simulink model "syncbuck_CL"  (Simulink 7.5)
settings: Solver=ode45  StartTime=0.0  StopTime=200e-6  MaxStep=0.1e-6  RelTol=1e-3
libraries: simulink x1
settings Model: Creator=Dragan Maksimovic  LastModifiedBy=Dragan Maksimovic

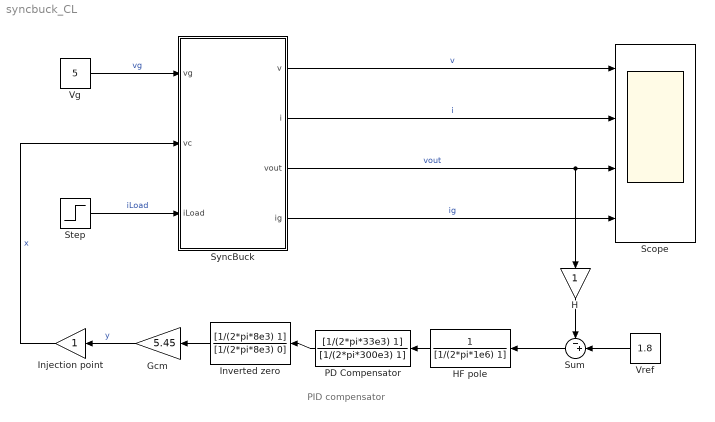
== system syncbuck_CL ==
  note: PID compensator
  " Inverted zero" : TransferFcn  Numerator=[1/(2*pi*8e3) 1]  Denominator=[1/(2*pi*8e3) 0]
  Gcm : Gain  Gain=5.45  ParameterDataType=fixdt(1, 16)  ParameterScaling=2^0  OutDataType=fixdt(1, 16)  OutScaling=2^0
  H : Gain  ParameterDataType=fixdt(1, 16)  ParameterScaling=2^0  OutDataType=fixdt(1, 16)  OutScaling=2^0
  HF pole : TransferFcn  Denominator=[1/(2*pi*1e6) 1]
  Injection point : Gain  ParameterDataType=fixdt(1, 16)  ParameterScaling=2^0  OutDataType=fixdt(1, 16)  OutScaling=2^0
  PD Compensator : TransferFcn  Numerator=[1/(2*pi*33e3) 1]  Denominator=[1/(2*pi*300e3) 1]
  Scope : Scope  NumInputPorts=4
      settings: TimeRange=3.000131492439188e-005  YMin=1.74~-5~1.74~-5  YMax=1.84~10~1.84~10
  Step : Step  Time=120e-6  After=5  SampleTime=0
  Sum : Sum  Inputs=-+|  OutDataType=fixdt(1, 16)  OutScaling=2^0
  SyncBuck : Subsystem  mask{L=1e-6, i0=0, C=200e-6, v0=1.8, fs=1e6, VM=1, Ron1=20e-3, Ron2=20e-3, RL=10e-3, Resr=0.8e-3, sw=off}
      mask prompts: L "Inductance L"; i0 "Initial inductor current i(0)"; C "Capacitance C"; v0 "Initial capacitor voltage v(0)"; fs "Switching frequency fs"; VM "PWM ramp amplitude VM"; Ron1 "Transistor switch Ron1"; Ron2 "Sync rectifier switch Ron2"; RL "Inductor resistance RL"; Resr "Capacitor esr Resr"; sw "Switching model?"
  Vg : Constant  Value=5  OutDataType=fixdt(1, 16)  OutScaling=2^0
  Vref : Constant  Value=1.8  OutDataType=fixdt(1, 16)  OutScaling=2^0
  wires:
  Vg/1 -> SyncBuck/1(vg)  "vg"
  Step/1 -> SyncBuck/3(iLoad)  "iLoad"
  SyncBuck/1(v) -> Scope/1  "v"
  SyncBuck/2(i) -> Scope/2  "i"
  SyncBuck/3(vout) -> Scope/3, H/1  "vout"
  SyncBuck/4(ig) -> Scope/4  "ig"
  Vref/1 -> Sum/2
  Injection point/1 -> SyncBuck/2(vc)  "x"
  H/1 -> Sum/1
  PD Compensator/1 -> " Inverted zero"/1
  " Inverted zero"/1 -> Gcm/1
  Gcm/1 -> Injection point/1  "y"
  Sum/1 -> HF pole/1
  HF pole/1 -> PD Compensator/1

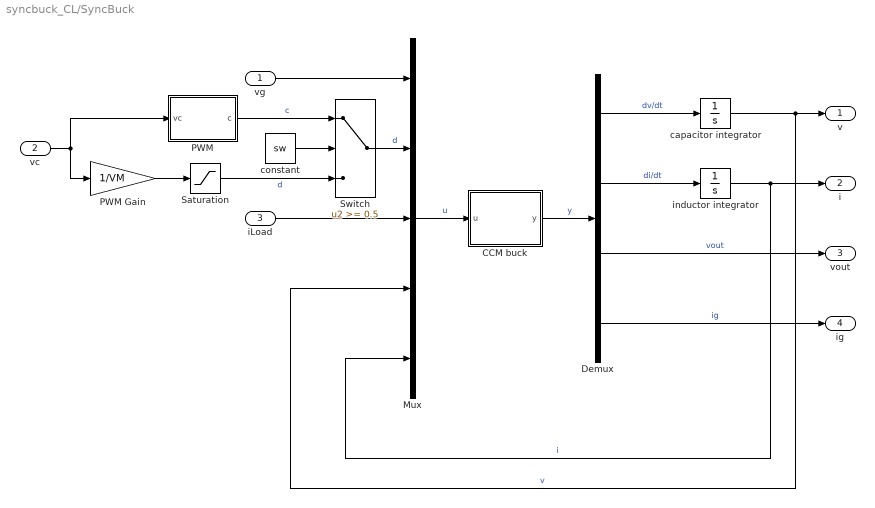
== system syncbuck_CL/SyncBuck ==
  vg : Inport  OutDataType=fixdt(1, 16)  OutScaling=2^0
  vc : Inport  Port=2  OutDataType=fixdt(1, 16)  OutScaling=2^0
  iLoad : Inport  Port=3  OutDataType=fixdt(1, 16)  OutScaling=2^0
  CCM buck : Stateflow chart  TreatAsAtomicUnit=on
  Demux : Demux
  Mux : Mux  Inputs=5
  PWM : Subsystem
  PWM Gain : Gain  Gain=1/VM  ParameterDataType=fixdt(1, 16)  ParameterScaling=2^0  OutDataType=fixdt(1, 16)  OutScaling=2^0
  Saturation : Saturate  UpperLimit=1  LowerLimit=0  OutDataType=fixdt(1, 16)  OutScaling=2^0
  Switch : Switch  Threshold=0.5  OutDataType=fixdt(1, 16)  OutScaling=2^0
  capacitor integrator : Integrator  InitialCondition=v0
  constant : Constant  Value=sw  OutDataType=fixdt(1, 16)  OutScaling=2^0
  inductor integrator : Integrator  InitialCondition=i0
  v : Outport  OutDataType=fixdt(1, 16)  OutScaling=2^0
  i : Outport  Port=2  OutDataType=fixdt(1, 16)  OutScaling=2^0
  vout : Outport  Port=3  OutDataType=fixdt(1, 16)  OutScaling=2^0
  ig : Outport  Port=4  OutDataType=fixdt(1, 16)  OutScaling=2^0
  wires:
  Demux/1 -> capacitor integrator/1  "dv/dt"
  capacitor integrator/1 -> v/1, Mux/4  "v"
  inductor integrator/1 -> i/1, Mux/5  "i"
  Demux/2 -> inductor integrator/1  "di/dt"
  Demux/3 -> vout/1  "vout"
  Demux/4 -> ig/1  "ig"
  CCM buck/1(y) -> Demux/1  "y"
  vg/1 -> Mux/1
  iLoad/1 -> Mux/3
  Mux/1 -> CCM buck/1(u)  "u"
  Switch/1 -> Mux/2  "d"
  constant/1 -> Switch/2
  vc/1 -> PWM/1(vc), PWM Gain/1
  PWM/1(c) -> Switch/1  "c"
  PWM Gain/1 -> Saturation/1
  Saturation/1 -> Switch/3  "d"

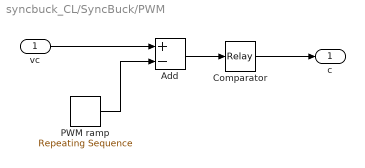
== system syncbuck_CL/SyncBuck/PWM ==
  vc : Inport  OutDataType=fixdt(1, 16)  OutScaling=2^0
  Add : Sum  Inputs=+-  OutDataType=fixdt(1, 16)  OutScaling=2^-10
  Comparator : Relay  OutDataType=fixdt(1, 16)  OutScaling=2^0
  PWM ramp : simulink/Sources/Repeating Sequence  SystemSampleTime=-1  rep_seq_t=[0 1/fs]  rep_seq_y=[0 VM]
  c : Outport  OutDataType=fixdt(1, 16)  OutScaling=2^0
  wires:
  vc/1 -> Add/1
  PWM ramp/1 -> Add/2
  Add/1 -> Comparator/1
  Comparator/1 -> c/1

== matlab function SyncBuck/CCM buck ==
  data: u input double size=5; y output double; L parameter double; C parameter double; RL parameter double; Ron1 parameter double; Ron2 parameter double; Resr parameter double
function y = CCMbuck(u,L,C,RL,Ron1,Ron2,Resr)
% State equations of a synchronous buck converter
% Conduction losses due to RL, Ron1, Ron2, Resr are included
% Inputs: u = [vg d iLoad v i]
% Outputs: y = [iC/C vL/L vout ig]
% Parameters: L, C, RL, Ron1, Ron2, Resr
%
% variables
vg = u(1); % input voltage
d = u(2); % switch control d=c (in the switching model), d in the averaged model
iLoad = u(3); % load current
v = u(4); % capacitor voltage
i = u(5); % inductor current
%
% state equations
vout = v + Resr*(i-iLoad); % output voltage
ig = d*i; % input current
iC = i - iLoad; % capacitor current
vL = d*(vg-(Ron1+RL)*i-vout)+(1-d)*(-(Ron2+RL)*i - vout); % inductor voltage
%
% output
y = [iC/C vL/L vout ig];
